simulink model "linealizado"  (R2021a)
settings: Solver=VariableStepAuto  StartTime=0.0  StopTime=120  RelTol=1e-3
values from neighbouring files (symbols this model uses):
  c_f = 800000    [engine_data.mat]
  c_T = 1    [engine_data.mat]
  sysd = c2d(sysc, Ts_1)    [linealizacion_0.m]
  Ts_1 = 0.1    [linealizacion_0.m]
  Tstart = 5    [engine_data.mat]
libraries: pid_lib x3, mpclib x1
settings Model: Creator=Seb  LastModifiedBy=Seb

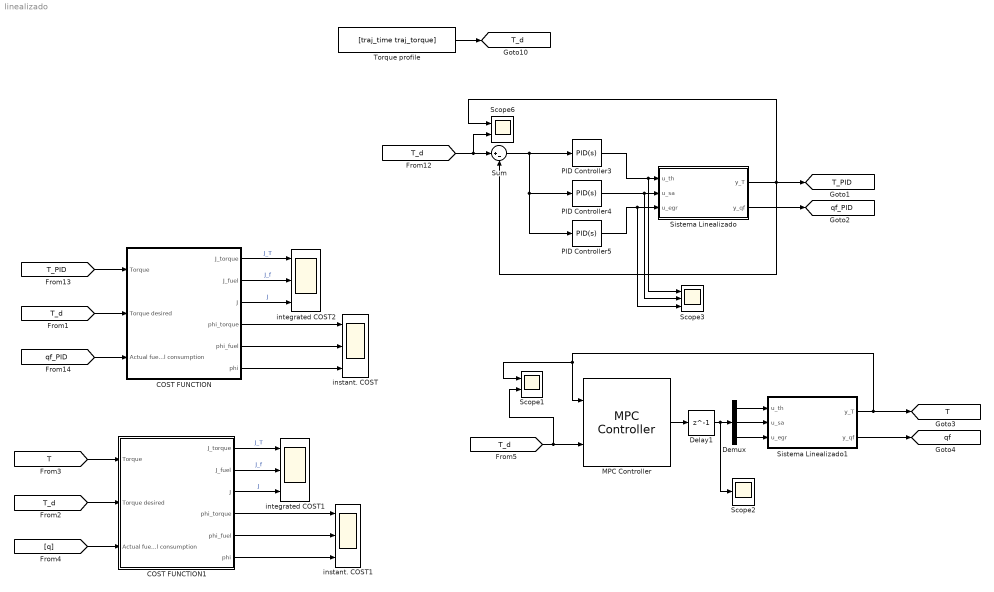
== system linealizado ==
  COST FUNCTION : Subsystem
  COST FUNCTION1 : Subsystem
  Delay1 : Delay  DelayLength=1  InitialCondition=0  SampleTime=0.001
  Demux : Demux  Outputs=3
  MPC Controller : mpclib/MPC Controller  SCDEnableBlockLinearizationSpecification=on  mpcobj=mpc_1  is_multiple=0  enable_value=0  return_u0=off  updateMPCinCallerWorkspace=on  md_inport=off  mv_inport=off  uref_inport=off  return_cost=off  return_mvseq=off  return_qpstatus=off  return_xseq=off  return_state=off  return_ovseq=off  state_inport=off  umin_inport=off  umax_inport=off  ymin_inport=off  ymax_inport=off  cc_inport=off  ywt_inport=off  uwt_inport=off  duwt_inport=off  rhoeps_inport=off  pm_inport=off  MaximumP=10  HorizonChoice=FixedHorizon  n_ts=0.1  n_p=10  n_mv=3  n_md=0  n_ud=0  n_mo=1  n_uo=0  BlockDataType=double  SampleTimeInherited=off  switch_inport=off
  PID Controller3 : pid_lib/PID Controller  Controller=PID  Form=Parallel  TimeDomain=Continuous-time  UseExternalTs=off  SampleTime=-1  IntegratorMethod=Forward Euler  FilterMethod=Forward Euler  ControllerParametersSource=internal  P=0.15  I=0.75  D=0  UseFilter=on  N=100  TunerSelectOption=Transfer Function Based (PID Tuner App)  InitialConditionSource=internal  InitialConditionForIntegrator=0  InitialConditionForFilter=0  DifferentiatorICPrevScaledInput=0  ExternalReset=none  TrackingMode=off  Kt=1  LimitOutput=off  SatLimitsSource=internal  UpperSaturationLimit=inf  LowerSaturationLimit=-inf  LinearizeAsGain=on  AntiWindupMode=none  Kb=1  POutMin=[]  POutMax=[]  IOutMin=[]  IOutMax=[]  DOutMin=[]  DOutMax=[]  NOutMin=[]  NOutMax=[]  SumOutMin=[]  SumOutMax=[]  SaturationOutMin=[]  SaturationOutMax=[]  PParamMin=[]  PParamMax=[]  IParamMin=[]  IParamMax=[]  DParamMin=[]  DParamMax=[]  NParamMin=[]  NParamMax=[]  KbParamMin=[]  KbParamMax=[]  KtParamMin=[]  KtParamMax=[]  KbOutMin=[]  KbOutMax=[]  KtOutMin=[]  KtOutMax=[]  IntegratorOutMin=[]  IntegratorOutMax=[]  FilterOutMin=[]  FilterOutMax=[]  SumI1OutMin=[]  SumI1OutMax=[]  SumI2OutMin=[]  SumI2OutMax=[]  SumI3OutMin=[]  SumI3OutMax=[]  SumI4OutMin=[]  SumI4OutMax=[]  SumDOutMin=[]  SumDOutMax=[]  DifferentiatorOutMin=[]  DifferentiatorOutMax=[]  FilterDiffOutCoefMin=[]  FilterDiffOutCoefMax=[]  ReciprocalOutMin=[]  ReciprocalOutMax=[]  SumDenOutMin=[]  SumDenOutMax=[]  SumNumOutMin=[]  SumNumOutMax=[]  DivideOutMin=[]  DivideOutMax=[]  UdiffTsProdOutMin=[]  UdiffTsProdOutMax=[]  NTsProdOutMin=[]  NTsProdOutMax=[]  UintegralTsProdOutMin=[]  UintegralTsProdOutMax=[]  UngainTsProdOutMin=[]  UngainTsProdOutMax=[]  IntegratorContinuousStateAttributes=''  IntegratorStateMustResolveToSignalObject=off  IntegratorRTWStateStorageClass=Auto  FilterContinuousStateAttributes=''  FilterStateMustResolveToSignalObject=off  FilterRTWStateStorageClass=Auto  ParallelPVariant=InternalParameters  IdealPVariant=Disabled  IVariant=InternalParameters  DVariant=InternalParameters  IntegratorVariant=Continuous  SatVariant=Disabled  AWVariant=Passthrough  PCopyVariant=Disabled  TRVariant=Disabled  FdbkBlocksVariant=Forward  IdealPFdbkVariant=Disabled  SatFdbkVariant=Disabled  DerivativeFilterVariant=ContFilter  NVariant=InternalParameters  NCopyVariant=Disabled  FilterICVariant=InternalICsFilter  IntegratorICVariant=InternalICs  ExternalResetVariant=Disabled  TRSumVariant=Passthrough  SumFdbkVariant=Disabled  SumVariant=Sum_PID  TsampFilterVariant=InternalTs  TsampNgainVariant=Passthrough  TsampIntegralVariant=Passthrough  ExternalSaturationOutDataTypeStr=Inherit: Same as second input
  PID Controller4 : pid_lib/PID Controller  Controller=PID  Form=Parallel  TimeDomain=Continuous-time  UseExternalTs=off  SampleTime=-1  IntegratorMethod=Forward Euler  FilterMethod=Forward Euler  ControllerParametersSource=internal  P=0.3  I=0.1  D=0  UseFilter=on  N=100  TunerSelectOption=Transfer Function Based (PID Tuner App)  InitialConditionSource=internal  InitialConditionForIntegrator=0  InitialConditionForFilter=0  DifferentiatorICPrevScaledInput=0  ExternalReset=none  TrackingMode=off  Kt=1  LimitOutput=off  SatLimitsSource=internal  UpperSaturationLimit=inf  LowerSaturationLimit=-inf  LinearizeAsGain=on  AntiWindupMode=none  Kb=1  POutMin=[]  POutMax=[]  IOutMin=[]  IOutMax=[]  DOutMin=[]  DOutMax=[]  NOutMin=[]  NOutMax=[]  SumOutMin=[]  SumOutMax=[]  SaturationOutMin=[]  SaturationOutMax=[]  PParamMin=[]  PParamMax=[]  IParamMin=[]  IParamMax=[]  DParamMin=[]  DParamMax=[]  NParamMin=[]  NParamMax=[]  KbParamMin=[]  KbParamMax=[]  KtParamMin=[]  KtParamMax=[]  KbOutMin=[]  KbOutMax=[]  KtOutMin=[]  KtOutMax=[]  IntegratorOutMin=[]  IntegratorOutMax=[]  FilterOutMin=[]  FilterOutMax=[]  SumI1OutMin=[]  SumI1OutMax=[]  SumI2OutMin=[]  SumI2OutMax=[]  SumI3OutMin=[]  SumI3OutMax=[]  SumI4OutMin=[]  SumI4OutMax=[]  SumDOutMin=[]  SumDOutMax=[]  DifferentiatorOutMin=[]  DifferentiatorOutMax=[]  FilterDiffOutCoefMin=[]  FilterDiffOutCoefMax=[]  ReciprocalOutMin=[]  ReciprocalOutMax=[]  SumDenOutMin=[]  SumDenOutMax=[]  SumNumOutMin=[]  SumNumOutMax=[]  DivideOutMin=[]  DivideOutMax=[]  UdiffTsProdOutMin=[]  UdiffTsProdOutMax=[]  NTsProdOutMin=[]  NTsProdOutMax=[]  UintegralTsProdOutMin=[]  UintegralTsProdOutMax=[]  UngainTsProdOutMin=[]  UngainTsProdOutMax=[]  IntegratorContinuousStateAttributes=''  IntegratorStateMustResolveToSignalObject=off  IntegratorRTWStateStorageClass=Auto  FilterContinuousStateAttributes=''  FilterStateMustResolveToSignalObject=off  FilterRTWStateStorageClass=Auto  ParallelPVariant=InternalParameters  IdealPVariant=Disabled  IVariant=InternalParameters  DVariant=InternalParameters  IntegratorVariant=Continuous  SatVariant=Disabled  AWVariant=Passthrough  PCopyVariant=Disabled  TRVariant=Disabled  FdbkBlocksVariant=Forward  IdealPFdbkVariant=Disabled  SatFdbkVariant=Disabled  DerivativeFilterVariant=ContFilter  NVariant=InternalParameters  NCopyVariant=Disabled  FilterICVariant=InternalICsFilter  IntegratorICVariant=InternalICs  ExternalResetVariant=Disabled  TRSumVariant=Passthrough  SumFdbkVariant=Disabled  SumVariant=Sum_PID  TsampFilterVariant=InternalTs  TsampNgainVariant=Passthrough  TsampIntegralVariant=Passthrough  ExternalSaturationOutDataTypeStr=Inherit: Same as second input
  PID Controller5 : pid_lib/PID Controller  Controller=PID  Form=Parallel  TimeDomain=Continuous-time  UseExternalTs=off  SampleTime=-1  IntegratorMethod=Forward Euler  FilterMethod=Forward Euler  ControllerParametersSource=internal  P=0  I=0  D=0  UseFilter=on  N=100  TunerSelectOption=Transfer Function Based (PID Tuner App)  InitialConditionSource=internal  InitialConditionForIntegrator=0  InitialConditionForFilter=0  DifferentiatorICPrevScaledInput=0  ExternalReset=none  TrackingMode=off  Kt=1  LimitOutput=off  SatLimitsSource=internal  UpperSaturationLimit=inf  LowerSaturationLimit=-inf  LinearizeAsGain=on  AntiWindupMode=none  Kb=1  POutMin=[]  POutMax=[]  IOutMin=[]  IOutMax=[]  DOutMin=[]  DOutMax=[]  NOutMin=[]  NOutMax=[]  SumOutMin=[]  SumOutMax=[]  SaturationOutMin=[]  SaturationOutMax=[]  PParamMin=[]  PParamMax=[]  IParamMin=[]  IParamMax=[]  DParamMin=[]  DParamMax=[]  NParamMin=[]  NParamMax=[]  KbParamMin=[]  KbParamMax=[]  KtParamMin=[]  KtParamMax=[]  KbOutMin=[]  KbOutMax=[]  KtOutMin=[]  KtOutMax=[]  IntegratorOutMin=[]  IntegratorOutMax=[]  FilterOutMin=[]  FilterOutMax=[]  SumI1OutMin=[]  SumI1OutMax=[]  SumI2OutMin=[]  SumI2OutMax=[]  SumI3OutMin=[]  SumI3OutMax=[]  SumI4OutMin=[]  SumI4OutMax=[]  SumDOutMin=[]  SumDOutMax=[]  DifferentiatorOutMin=[]  DifferentiatorOutMax=[]  FilterDiffOutCoefMin=[]  FilterDiffOutCoefMax=[]  ReciprocalOutMin=[]  ReciprocalOutMax=[]  SumDenOutMin=[]  SumDenOutMax=[]  SumNumOutMin=[]  SumNumOutMax=[]  DivideOutMin=[]  DivideOutMax=[]  UdiffTsProdOutMin=[]  UdiffTsProdOutMax=[]  NTsProdOutMin=[]  NTsProdOutMax=[]  UintegralTsProdOutMin=[]  UintegralTsProdOutMax=[]  UngainTsProdOutMin=[]  UngainTsProdOutMax=[]  IntegratorContinuousStateAttributes=''  IntegratorStateMustResolveToSignalObject=off  IntegratorRTWStateStorageClass=Auto  FilterContinuousStateAttributes=''  FilterStateMustResolveToSignalObject=off  FilterRTWStateStorageClass=Auto  ParallelPVariant=InternalParameters  IdealPVariant=Disabled  IVariant=InternalParameters  DVariant=InternalParameters  IntegratorVariant=Continuous  SatVariant=Disabled  AWVariant=Passthrough  PCopyVariant=Disabled  TRVariant=Disabled  FdbkBlocksVariant=Forward  IdealPFdbkVariant=Disabled  SatFdbkVariant=Disabled  DerivativeFilterVariant=ContFilter  NVariant=InternalParameters  NCopyVariant=Disabled  FilterICVariant=InternalICsFilter  IntegratorICVariant=InternalICs  ExternalResetVariant=Disabled  TRSumVariant=Passthrough  SumFdbkVariant=Disabled  SumVariant=Sum_PID  TsampFilterVariant=InternalTs  TsampNgainVariant=Passthrough  TsampIntegralVariant=Passthrough  ExternalSaturationOutDataTypeStr=Inherit: Same as second input
  Scope1 : Scope  NumInputPorts=2
  Scope2 : Scope
  Scope3 : Scope  NumInputPorts=3
  Scope6 : Scope  NumInputPorts=2
  Sistema Linealizado : Subsystem
  Sistema Linealizado1 : Subsystem
  Sum : Sum  Inputs=|+-
  Torque profile : FromWorkspace  VariableName=[traj_time traj_torque]  SampleTime=-1  OutputAfterFinalValue=Holding final value
  instant. COST : Scope  NumInputPorts=3
  instant. COST1 : Scope  NumInputPorts=3
  integrated COST1 : Scope  NumInputPorts=3
  integrated COST2 : Scope  NumInputPorts=3
  tag scope: T=global, T_PID=global, T_d=global, qf=global, qf_PID=global
  wires:
  Torque profile/1 -> [T_d]
  [T_d] -> Scope6/2, Sum/1
  PID Controller4/1 -> Scope3/2, Sistema Linealizado/2(u_sa)
  PID Controller3/1 -> Scope3/1, Sistema Linealizado/1(u_th)
  PID Controller5/1 -> Scope3/3, Sistema Linealizado/3(u_egr)
  Sum/1 -> PID Controller3/1, PID Controller4/1, PID Controller5/1
  Sistema Linealizado/1(y_T) -> [T_PID], Scope6/1, Sum/2
  COST FUNCTION/4(phi_torque) -> instant. COST/1
  COST FUNCTION/1(J_torque) -> integrated COST2/1  "J_T"
  COST FUNCTION/2(J_fuel) -> integrated COST2/2  "J_f"
  COST FUNCTION/5(phi_fuel) -> instant. COST/2
  [qf_PID] -> COST FUNCTION/3(Actual fuel consumption)
  COST FUNCTION/6(phi) -> instant. COST/3
  [T_d] -> COST FUNCTION/2(Torque desired)
  [T_PID] -> COST FUNCTION/1(Torque)
  COST FUNCTION/3(J) -> integrated COST2/3  "J"
  Sistema Linealizado/2(y_qf) -> [qf_PID]
  COST FUNCTION1/3(J) -> integrated COST1/3  "J"
  [T] -> COST FUNCTION1/1(Torque)
  [T_d] -> COST FUNCTION1/2(Torque desired)
  COST FUNCTION1/6(phi) -> instant. COST1/3
  [q] -> COST FUNCTION1/3(Actual fuel consumption)
  COST FUNCTION1/5(phi_fuel) -> instant. COST1/2
  COST FUNCTION1/2(J_fuel) -> integrated COST1/2  "J_f"
  COST FUNCTION1/1(J_torque) -> integrated COST1/1  "J_T"
  COST FUNCTION1/4(phi_torque) -> instant. COST1/1
  MPC Controller/1 -> Delay1/1
  Demux/1 -> Sistema Linealizado1/1(u_th)
  Demux/2 -> Sistema Linealizado1/2(u_sa)
  Demux/3 -> Sistema Linealizado1/3(u_egr)
  [T_d] -> Scope1/2, MPC Controller/2
  Sistema Linealizado1/2(y_qf) -> [qf]
  Sistema Linealizado1/1(y_T) -> Scope1/1, MPC Controller/1, [T]
  Delay1/1 -> Scope2/1, Demux/1

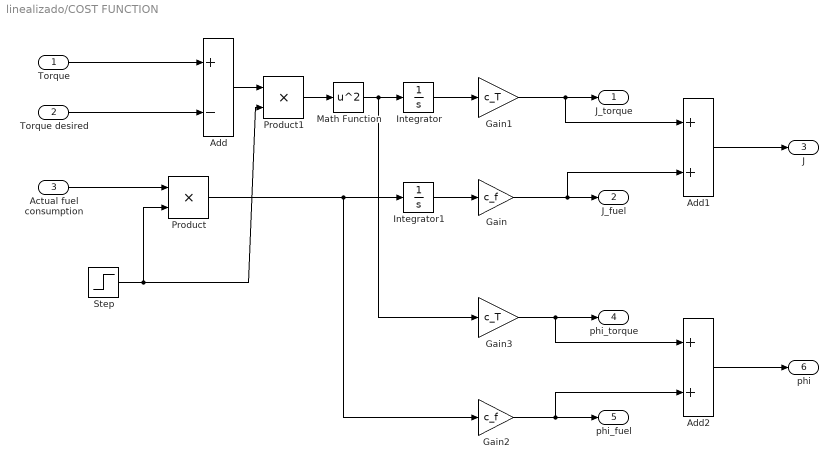
== system linealizado/COST FUNCTION ==
  Torque : Inport
  Torque desired : Inport  Port=2
  Actual fuel consumption : Inport  Port=3
  Add : Sum  Inputs=+-
  Add1 : Sum
  Add2 : Sum
  Gain : Gain  Gain=c_f
  Gain1 : Gain  Gain=c_T
  Gain2 : Gain  Gain=c_f
  Gain3 : Gain  Gain=c_T
  Integrator : Integrator
  Integrator1 : Integrator
  Math Function : Math  Operator=square  SignedPower=on  SaturateOnIntegerOverflow=on
  Product : Product
  Product1 : Product
  Step : Step  Time=Tstart  SampleTime=0
  J_torque : Outport
  J_fuel : Outport  Port=2
  J : Outport  Port=3
  phi_torque : Outport  Port=4
  phi_fuel : Outport  Port=5
  phi : Outport  Port=6
  wires:
  Torque/1 -> Add/1
  Torque desired/1 -> Add/2
  Gain/1 -> Add1/2, J_fuel/1
  Gain1/1 -> Add1/1, J_torque/1
  Math Function/1 -> Gain3/1, Integrator/1
  Integrator/1 -> Gain1/1
  Actual fuel consumption/1 -> Product/1
  Product/1 -> Gain2/1, Integrator1/1
  Step/1 -> Product1/2, Product/2
  Add/1 -> Product1/1
  Product1/1 -> Math Function/1
  Add1/1 -> J/1
  Integrator1/1 -> Gain/1
  Gain3/1 -> phi_torque/1, Add2/1
  Add2/1 -> phi/1
  Gain2/1 -> Add2/2, phi_fuel/1

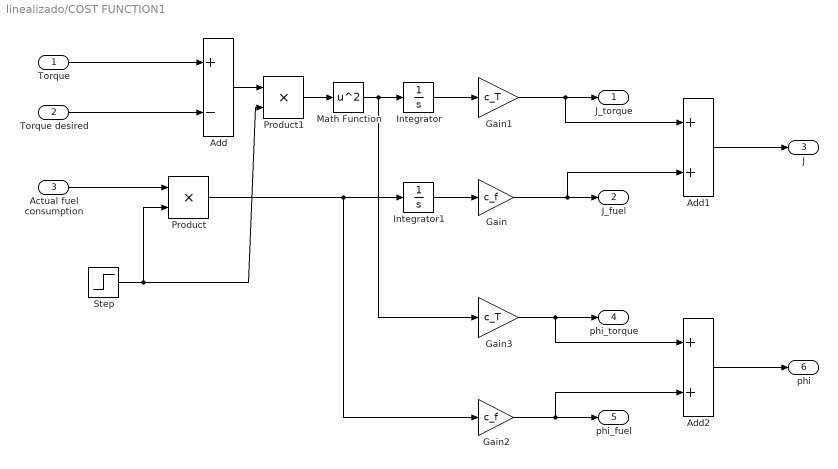
== system linealizado/COST FUNCTION1 ==
  Torque : Inport
  Torque desired : Inport  Port=2
  Actual fuel consumption : Inport  Port=3
  Add : Sum  Inputs=+-
  Add1 : Sum
  Add2 : Sum
  Gain : Gain  Gain=c_f
  Gain1 : Gain  Gain=c_T
  Gain2 : Gain  Gain=c_f
  Gain3 : Gain  Gain=c_T
  Integrator : Integrator
  Integrator1 : Integrator
  Math Function : Math  Operator=square  SignedPower=on  SaturateOnIntegerOverflow=on
  Product : Product
  Product1 : Product
  Step : Step  Time=Tstart  SampleTime=0
  J_torque : Outport
  J_fuel : Outport  Port=2
  J : Outport  Port=3
  phi_torque : Outport  Port=4
  phi_fuel : Outport  Port=5
  phi : Outport  Port=6
  wires:
  Gain2/1 -> phi_fuel/1, Add2/2
  Add2/1 -> phi/1
  Gain3/1 -> Add2/1, phi_torque/1
  Integrator1/1 -> Gain/1
  Add1/1 -> J/1
  Product1/1 -> Math Function/1
  Add/1 -> Product1/1
  Step/1 -> Product/2, Product1/2
  Product/1 -> Integrator1/1, Gain2/1
  Actual fuel consumption/1 -> Product/1
  Integrator/1 -> Gain1/1
  Math Function/1 -> Integrator/1, Gain3/1
  Gain1/1 -> J_torque/1, Add1/1
  Gain/1 -> J_fuel/1, Add1/2
  Torque desired/1 -> Add/2
  Torque/1 -> Add/1

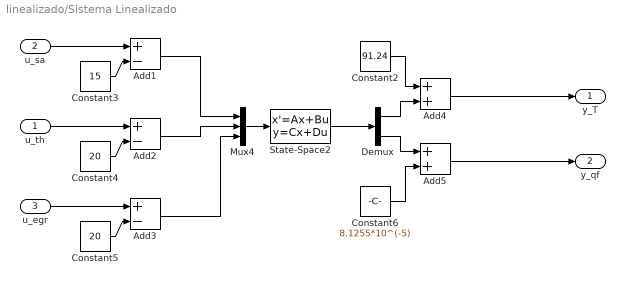
== system linealizado/Sistema Linealizado ==
  u_th : Inport
  u_sa : Inport  Port=2
  u_egr : Inport  Port=3
  Add1 : Sum  Inputs=+-
  Add2 : Sum  Inputs=+-
  Add3 : Sum  Inputs=+-
  Add4 : Sum
  Add5 : Sum
  Constant2 : Constant  Value=91.24
  Constant3 : Constant  Value=15
  Constant4 : Constant  Value=20
  Constant5 : Constant  Value=20
  Constant6 : Constant  Value=8.1255*10^(-5)
  Demux : Demux  Outputs=2
  Mux4 : Mux  Inputs=3
  State-Space2 : StateSpace  A=[0]  B=[0 0 0]  C=[0;0]  D=[0.1577 6.775 0.2081; 5.8115*10^(-12) 4.289*10^(-6) 1.4775*10^(-8)]  InitialCondition=0
  y_T : Outport
  y_qf : Outport  Port=2
  wires:
  u_sa/1 -> Add1/1
  Constant3/1 -> Add1/2
  Constant2/1 -> Add4/1
  State-Space2/1 -> Demux/1
  Demux/1 -> Add4/2
  Add3/1 -> Mux4/3
  Constant5/1 -> Add3/2
  Mux4/1 -> State-Space2/1
  Add1/1 -> Mux4/1
  Add2/1 -> Mux4/2
  Constant6/1 -> Add5/2
  Constant4/1 -> Add2/2
  Demux/2 -> Add5/1
  Add5/1 -> y_qf/1
  u_egr/1 -> Add3/1
  u_th/1 -> Add2/1
  Add4/1 -> y_T/1

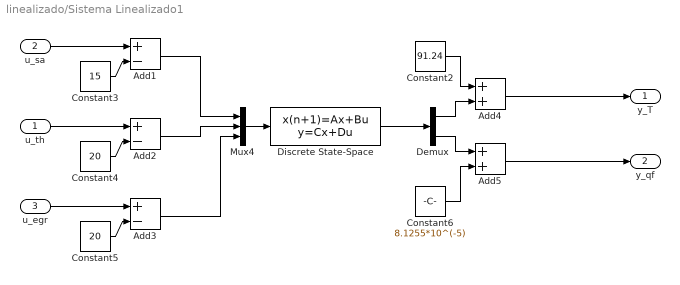
== system linealizado/Sistema Linealizado1 ==
  u_th : Inport
  u_sa : Inport  Port=2
  u_egr : Inport  Port=3
  Add1 : Sum  Inputs=+-
  Add2 : Sum  Inputs=+-
  Add3 : Sum  Inputs=+-
  Add4 : Sum
  Add5 : Sum
  Constant2 : Constant  Value=91.24
  Constant3 : Constant  Value=15
  Constant4 : Constant  Value=20
  Constant5 : Constant  Value=20
  Constant6 : Constant  Value=8.1255*10^(-5)
  Demux : Demux  Outputs=2
  Discrete State-Space : DiscreteStateSpace  A=sysd.A  B=sysd.B  C=sysd.C  D=sysd.D  SampleTime=Ts_1
  Mux4 : Mux  Inputs=3
  y_T : Outport
  y_qf : Outport  Port=2
  wires:
  Add4/1 -> y_T/1
  u_th/1 -> Add2/1
  u_egr/1 -> Add3/1
  Add5/1 -> y_qf/1
  Demux/2 -> Add5/1
  Constant4/1 -> Add2/2
  Constant6/1 -> Add5/2
  Add2/1 -> Mux4/2
  Add1/1 -> Mux4/1
  Mux4/1 -> Discrete State-Space/1
  Constant5/1 -> Add3/2
  Add3/1 -> Mux4/3
  Demux/1 -> Add4/2
  Discrete State-Space/1 -> Demux/1
  Constant2/1 -> Add4/1
  Constant3/1 -> Add1/2
  u_sa/1 -> Add1/1
